simulink model "EM25_Matlab"  (R2024b)
settings: Solver=FixedStepAuto  StartTime=0.0  StopTime=0.5  RelTol=1e-3
libraries: spsRMSLib x10, spsThreePhaseVIMeasurementLib x6, spsGroundLib x6, spsThreePhaseTransformerTwoWindingsLib x5, eePowerMeasurement x5, spsThreePhaseParallelRLCBranchLib x4, spsThreePhaseBreakerLib x4, spsSynchronousMachinepuStandardLib x3, spsThreePhasePISectionLineLib x1, spsThreePhaseSeriesRLCLoadLib x1, sps_lib x1
settings Model: Creator=User  LastModifiedBy=User

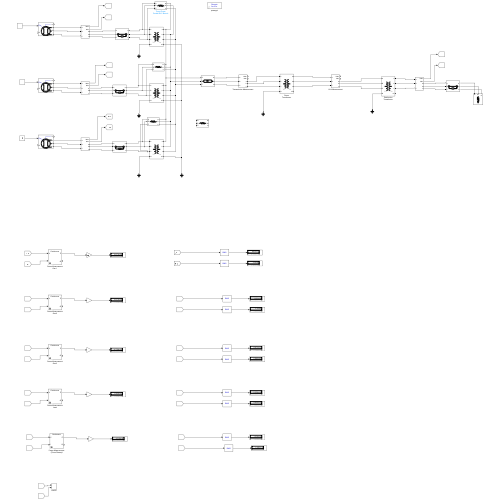
[thumbnail: Simulink's stored preview of the top-level diagram]
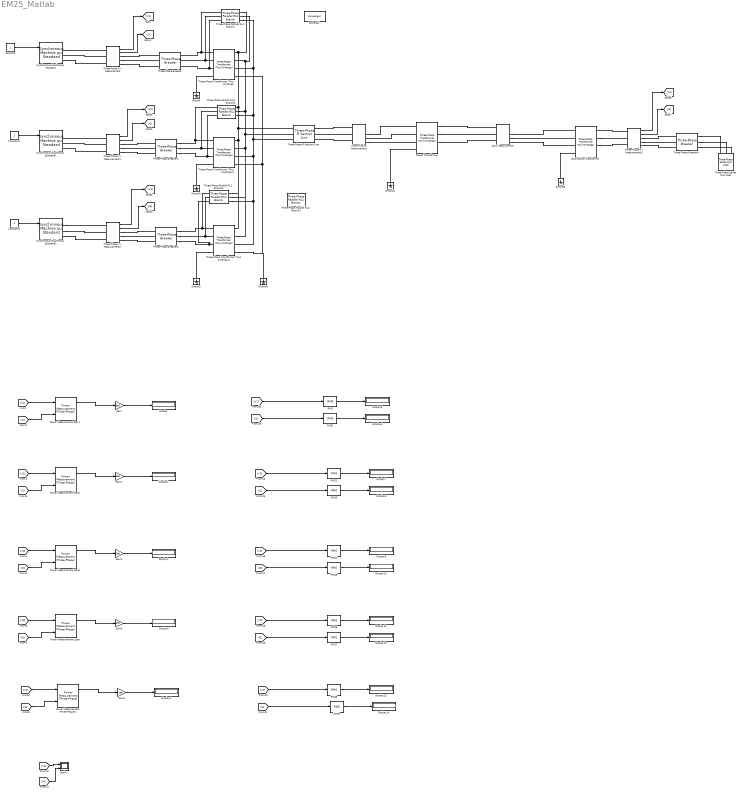
== system EM25_Matlab ==
  11kV Measurement : spsThreePhaseVIMeasurementLib/Three-Phase V-I Measurement  VoltageMeasurement=phase-to-ground  SetLabelV=off  LabelV=Vabc  Vpu=off  VpuLL=off  CurrentMeasurement=yes  SetLabelI=off  LabelI=Iabc  Ipu=off  Pbase=100e6  Vbase=500e3  OutputType=Complex  PhasorSimulation=off  PSBequivalent=0
  Constant : Constant
  Constant1 : Constant
  Constant2 : Constant
  Display{,1..14} (15 alike) : Display
  Distribution Transformer : spsThreePhaseTransformerTwoWindingsLib/Three-Phase Transformer (Two Windings)  Winding1Connection=Yn  Winding2Connection=Yn  CoreType=Three single-phase transformers  SetSaturation=off  Hysteresis=off  DataFile='hysteresis'  SetInitialFlux=off  Measurements=None  UNITS=pu  NominalPower=[ 3e6 , 50 ]  Winding1=[ 11000 , 0.01 , 0.05 ]  Winding2=[ 400 , 0.01 , 0.05 ]  Rm=500  Lm=500  L0=0.5  Saturation=[ 0,0 ; 0.0024,1.2 ; 1.0,1.52 ]  InitialFluxes=[ 0.8 , -0.8 , 0.7 ]  BreakLoop=off  DiscreteSolver=Trapezoidal iterative  DataType=off  TransfoNumber=1
  Gain{,1..4} (5 alike) : Gain  Gain=1e6
  Ground{,1..5} (6 alike) : spsGroundLib/Ground  LConnTagsString=a
  Power Transformer : spsThreePhaseTransformerTwoWindingsLib/Three-Phase Transformer (Two Windings)  Winding1Connection=Yn  Winding2Connection=Yn  CoreType=Three single-phase transformers  SetSaturation=off  Hysteresis=off  DataFile='hysteresis'  SetInitialFlux=off  Measurements=None  UNITS=pu  NominalPower=[ 10e6 , 50 ]  Winding1=[ 132000 , 0.002 , 0.08 ]  Winding2=[ 11000 , 0.002 , 0.08 ]  Rm=500  Lm=500  L0=0.5  Saturation=[ 0,0 ; 0.0024,1.2 ; 1.0,1.52 ]  InitialFluxes=[ 0.8 , -0.8 , 0.7 ]  BreakLoop=off  DiscreteSolver=Trapezoidal iterative  DataType=off  TransfoNumber=1
  Power Measurement (Three-Phase)4 : eePowerMeasurement/Power Measurement (Three-Phase)  LabelModeActiveChoice=Continuous  F=50  K=[0 1 2 3]  Seq=Positive  Ts=0
  Power Measurement Gen 1 : eePowerMeasurement/Power Measurement (Three-Phase)  LabelModeActiveChoice=Continuous  F=50  K=[0 1 2 3]  Seq=Positive  Ts=0
  Power Measurement Gen2 : eePowerMeasurement/Power Measurement (Three-Phase)  LabelModeActiveChoice=Continuous  F=50  K=[0 1 2 3]  Seq=Positive  Ts=0
  Power Measurement Gen3 : eePowerMeasurement/Power Measurement (Three-Phase)  LabelModeActiveChoice=Continuous  F=50  K=[0 1 2 3]  Seq=Positive  Ts=0
  Power Measurement Load : eePowerMeasurement/Power Measurement (Three-Phase)  LabelModeActiveChoice=Continuous  F=50  K=[0 1 2 3]  Seq=Positive  Ts=0
  RMS{,1..9} (10 alike) : spsRMSLib/RMS  TrueRMS=on  Freq=60  RMSInit=120  Ts=0
  Synchronous Machine pu Standard : spsSynchronousMachinepuStandardLib/Synchronous Machine pu Standard  PresetModel=No  MechanicalLoad=Mechanical power Pm  ShowDetailedParameters=on  RotorType=Round  Units=per unit standard parameters  MeasurementBus=off  NominalParameters=[1e6 11000 50]  Reactances1=[ 1.81, 0.3, 0.23, 1.76, 0.65, 0.25, 0.15 ]  Reactances2=[2.24 0.17 0.12 1.02 0.13 0.08]  dAxisTimeConstants=Short-circuit  qAxisTimeConstants=Short-circuit  TimeConstants1="[ 4.4849  0.0681  0.1  ]"  TimeConstants2=[ 8.0, 0.03, 1.0, 0.07 ]  TimeConstants3="[  4.49  0.0681  0.0513  ]"  TimeConstants4=[ 8.0, 0.03, 0.3371, 0.0295 ]  TimeConstants5=[ 1.01, 0.053, 0.1 ]  TimeConstants6=[ 1.3201, 0.023, 1.0, 0.07 ]  TimeConstants7=[0.012 0.003 0.003]  TimeConstants8=[ 1.3201, 0.0231, 0.3371, 0.0295 ]  StatorResistance=0.005  Mechanical=[3 0.01 2]  PolePairs=20  InitialConditions="[ 0  0  0  0  0  0  0  0  1 ]"  SetSaturation=off  Saturation=[0.6404,0.7127,0.8441,0.9214,0.9956,1.082,1.19,1.316,1.457;0.7,0.7698,0.8872,0.9466,0.9969,1.046,1.1,1.151,1.201]  LoadFlowParameters=[1,0,0,0,0]  TsPowergui=0  TsBlock=-1  IterativeModel=Trapezoidal non iterative  IterativeDiscreteModel=Trapezoidal non iterative  BusType=PV  Pref=0  Qref=0  Qmin=-inf  Qmax=inf  PLF=0  QLF=0
  Synchronous Machine pu Standard1 : spsSynchronousMachinepuStandardLib/Synchronous Machine pu Standard  PresetModel=No  MechanicalLoad=Mechanical power Pm  ShowDetailedParameters=on  RotorType=Round  Units=per unit standard parameters  MeasurementBus=off  NominalParameters=[2e6 12000 50]  Reactances1=[ 1.81, 0.3, 0.23, 1.76, 0.65, 0.25, 0.15 ]  Reactances2=[2.24 0.17 0.12 1.02 0.13 0.08]  dAxisTimeConstants=Short-circuit  qAxisTimeConstants=Short-circuit  TimeConstants1="[ 4.4849  0.0681  0.1  ]"  TimeConstants2=[ 8.0, 0.03, 1.0, 0.07 ]  TimeConstants3="[  4.49  0.0681  0.0513  ]"  TimeConstants4=[ 8.0, 0.03, 0.3371, 0.0295 ]  TimeConstants5=[ 1.01, 0.053, 0.1 ]  TimeConstants6=[ 1.3201, 0.023, 1.0, 0.07 ]  TimeConstants7=[0.012 0.003 0.003]  TimeConstants8=[ 1.3201, 0.0231, 0.3371, 0.0295 ]  StatorResistance=0.005  Mechanical=[3 0.01 2]  PolePairs=20  InitialConditions="[ 0  0  0  0  0  0  0  0  1 ]"  SetSaturation=off  Saturation=[0.6404,0.7127,0.8441,0.9214,0.9956,1.082,1.19,1.316,1.457;0.7,0.7698,0.8872,0.9466,0.9969,1.046,1.1,1.151,1.201]  LoadFlowParameters=[1,0,0,0,0]  TsPowergui=0  TsBlock=-1  IterativeModel=Trapezoidal non iterative  IterativeDiscreteModel=Trapezoidal non iterative  BusType=PV  Pref=0  Qref=0  Qmin=-inf  Qmax=inf  PLF=0  QLF=0
  Synchronous Machine pu Standard2 : spsSynchronousMachinepuStandardLib/Synchronous Machine pu Standard  PresetModel=No  MechanicalLoad=Mechanical power Pm  ShowDetailedParameters=on  RotorType=Round  Units=per unit standard parameters  MeasurementBus=off  NominalParameters=[4e6 10000 50]  Reactances1=[ 1.81, 0.3, 0.23, 1.76, 0.65, 0.25, 0.15 ]  Reactances2=[2.24 0.17 0.12 1.02 0.13 0.08]  dAxisTimeConstants=Short-circuit  qAxisTimeConstants=Short-circuit  TimeConstants1="[ 4.4849  0.0681  0.1  ]"  TimeConstants2=[ 8.0, 0.03, 1.0, 0.07 ]  TimeConstants3="[  4.49  0.0681  0.0513  ]"  TimeConstants4=[ 8.0, 0.03, 0.3371, 0.0295 ]  TimeConstants5=[ 1.01, 0.053, 0.1 ]  TimeConstants6=[ 1.3201, 0.023, 1.0, 0.07 ]  TimeConstants7=[0.012 0.003 0.003]  TimeConstants8=[ 1.3201, 0.0231, 0.3371, 0.0295 ]  StatorResistance=0.005  Mechanical=[3 0.01 2]  PolePairs=20  InitialConditions="[ 0  0  0  0  0  0  0  0  1 ]"  SetSaturation=off  Saturation=[0.6404,0.7127,0.8441,0.9214,0.9956,1.082,1.19,1.316,1.457;0.7,0.7698,0.8872,0.9466,0.9969,1.046,1.1,1.151,1.201]  LoadFlowParameters=[1,0,0,0,0]  TsPowergui=0  TsBlock=-1  IterativeModel=Trapezoidal non iterative  IterativeDiscreteModel=Trapezoidal non iterative  BusType=PV  Pref=0  Qref=0  Qmin=-inf  Qmax=inf  PLF=0  QLF=0
  Three-Phase PI Section Line : spsThreePhasePISectionLineLib/Three-Phase PI Section Line  LConnTagsString=a|b|c  RConnTagsString=A|B|C  Length=50  Frequency=50  Resistances=[ 0.05 0.15]  Inductances="[ 1e-3  3e-3]"  Capacitances=[1e-8 5e-9]
  Three-Phase Parallel RLC Branch{,1..3} (4 alike) : spsThreePhaseParallelRLCBranchLib/Three-Phase Parallel RLC Branch  LConnTagsString=A|B|C  RConnTagsString=A|B|C  BranchType=R  Resistance=1E6  Inductance=0  Capacitance=0  Measurements=None
  Three-Phase Series RLC Load : spsThreePhaseSeriesRLCLoadLib/Three-Phase Series RLC Load  LConnTagsString=A|B|C  Configuration=Y (grounded)  NominalVoltage=400  Vabc=[1e3 1e3 1e3]  Vabcp=[1e3 1e3 1e3]  NominalFrequency=50  UnbalancedPower=off  ActivePower=2e6  InductivePower=0  CapacitivePower=0  Pabc=[10e3 9e3 11e3]  QLabc=[100 90 110]  QCabc=[100 90 110]  Pabcp=[10e3 9e3 11e3]  QLabcp=[100 90 110]  QCabcp=[100 90 110]  Measurements=None  LoadType=constant Z
  Three-Phase Transformer (Two Windings) : spsThreePhaseTransformerTwoWindingsLib/Three-Phase Transformer (Two Windings)  Winding1Connection=Yn  Winding2Connection=Yn  CoreType=Three single-phase transformers  SetSaturation=off  Hysteresis=off  DataFile='hysteresis'  SetInitialFlux=off  Measurements=None  UNITS=pu  NominalPower=[ 1e6 , 50 ]  Winding1=[ 11000 , 0.002 , 0.08 ]  Winding2=[ 132000 , 0.002 , 0.08 ]  Rm=500  Lm=500  L0=0.5  Saturation=[ 0,0 ; 0.0024,1.2 ; 1.0,1.52 ]  InitialFluxes=[ 0.8 , -0.8 , 0.7 ]  BreakLoop=off  DiscreteSolver=Trapezoidal iterative  DataType=off  TransfoNumber=1
  Three-Phase Transformer (Two Windings)1 : spsThreePhaseTransformerTwoWindingsLib/Three-Phase Transformer (Two Windings)  Winding1Connection=Yn  Winding2Connection=Yn  CoreType=Three single-phase transformers  SetSaturation=off  Hysteresis=off  DataFile='hysteresis'  SetInitialFlux=off  Measurements=None  UNITS=pu  NominalPower=[ 2e6 , 50 ]  Winding1=[ 12000 , 0.002 , 0.08 ]  Winding2=[ 132000 , 0.002 , 0.08 ]  Rm=500  Lm=500  L0=0.5  Saturation=[ 0,0 ; 0.0024,1.2 ; 1.0,1.52 ]  InitialFluxes=[ 0.8 , -0.8 , 0.7 ]  BreakLoop=off  DiscreteSolver=Trapezoidal iterative  DataType=off  TransfoNumber=1
  Three-Phase Transformer (Two Windings)2 : spsThreePhaseTransformerTwoWindingsLib/Three-Phase Transformer (Two Windings)  Winding1Connection=Yn  Winding2Connection=Yn  CoreType=Three single-phase transformers  SetSaturation=off  Hysteresis=off  DataFile='hysteresis'  SetInitialFlux=off  Measurements=None  UNITS=pu  NominalPower=[ 4e6 , 50 ]  Winding1=[ 10000 , 0.002 , 0.08 ]  Winding2=[ 132000 , 0.002 , 0.08 ]  Rm=500  Lm=500  L0=0.5  Saturation=[ 0,0 ; 0.0024,1.2 ; 1.0,1.52 ]  InitialFluxes=[ 0.8 , -0.8 , 0.7 ]  BreakLoop=off  DiscreteSolver=Trapezoidal iterative  DataType=off  TransfoNumber=1
  Three-Phase V-I Measurement{,1..3} (4 alike) : spsThreePhaseVIMeasurementLib/Three-Phase V-I Measurement  VoltageMeasurement=phase-to-ground  SetLabelV=off  LabelV=Vabc  Vpu=off  VpuLL=off  CurrentMeasurement=yes  SetLabelI=off  LabelI=Iabc  Ipu=off  Pbase=100e6  Vbase=500e3  OutputType=Complex  PhasorSimulation=off  PSBequivalent=0
  Three-Phase Breaker{,1..2,4} (4 alike) : spsThreePhaseBreakerLib/Three-Phase Breaker  InitialState=closed  SwitchA=on  SwitchB=on  SwitchC=on  SwitchTimes="[1/60  5/60]"  External=off  BreakerResistance=0.001  SnubberResistance=1e5  SnubberCapacitance=inf  Measurements=None
  Transmission Measurement : spsThreePhaseVIMeasurementLib/Three-Phase V-I Measurement  VoltageMeasurement=phase-to-ground  SetLabelV=off  LabelV=Vabc  Vpu=off  VpuLL=off  CurrentMeasurement=yes  SetLabelI=off  LabelI=Iabc  Ipu=off  Pbase=100e6  Vbase=500e3  OutputType=Complex  PhasorSimulation=off  PSBequivalent=0
  load VI : Scope  NumInputPorts=2
  powergui : sps_lib/powergui  Priority=1  SimulationMode=Discrete  SampleTime=50e-6  frequency=60  Iterations=50  frequencyindice=50  Pbase=100e6  ErrMax=1e-4  UnitsV=kV  UnitsW=MW  buscounter=0  FunctionMessages=off  echomessages=off  EnableUseOfTLC=off  CurrentSourceSwitches=off  DisableSnubberDevices=off  DisableRonSwitches=off  DisableVfSwitches=off  DisplayEquations=off  AutomaticDiscreteSolvers=off  SolverType=Tustin/Backward Euler (TBE)  Interpol=off  ExternalGateDelay=off  methode=off  Ts=100  x0status=blocks  SPID=on  SwTol=0  HookPort=off  NonlinearTolerance=1e-4  nMaxIteration=100  ContinueOnMaxIteration=off  RestoreLinks=warning  ResistiveCurrentMeasurement=off  Frange=[0:2:500]  Ylog=off  Xlog=on  ShowGrid=off  save=off  variable=ZData  structure=0  ZoomFFT=off  StartTime=0.0  cycles=1  DisplayStyle=1  fundamental=60  FreqAxis=off  MaxFrequency=1000  frequencyindicesteady=1  RmsSteady=1  display=off
  wires:
  Constant/1 -> Synchronous Machine pu Standard/1
  Constant1/1 -> Synchronous Machine pu Standard1/1
  Constant2/1 -> Synchronous Machine pu Standard2/1
  Three-Phase V-I Measurement/1 -> [V1]
  Three-Phase V-I Measurement/2 -> [I1]
  Three-Phase V-I Measurement1/1 -> [V2]
  Three-Phase V-I Measurement1/2 -> [I2]
  Three-Phase V-I Measurement2/1 -> [V3]
  Three-Phase V-I Measurement2/2 -> [I3]
  [V1] -> Power Measurement Gen 1/1
  [I1] -> Power Measurement Gen 1/2
  Power Measurement Gen 1/1 -> Gain/1
  Gain/1 -> Display/1
  [V1] -> Power Measurement Gen2/1
  [I1] -> Power Measurement Gen2/2
  Gain1/1 -> Display1/1
  Power Measurement Gen2/1 -> Gain1/1
  [V2] -> Power Measurement Gen3/1
  [I2] -> Power Measurement Gen3/2
  Gain2/1 -> Display2/1
  Power Measurement Gen3/1 -> Gain2/1
  [V3] -> Power Measurement Load/1
  [I3] -> Power Measurement Load/2
  Gain3/1 -> Display3/1
  Power Measurement Load/1 -> Gain3/1
  [V4] -> Power Measurement (Three-Phase)4/1
  [I4] -> Power Measurement (Three-Phase)4/2
  Gain4/1 -> Display4/1
  Power Measurement (Three-Phase)4/1 -> Gain4/1
  Three-Phase V-I Measurement3/1 -> [V4]
  Three-Phase V-I Measurement3/2 -> [I4]
  [V4] -> load VI/1
  [I4] -> load VI/2
  [V1] -> RMS/1
  RMS/1 -> Display5/1
  [I1] -> RMS1/1
  RMS1/1 -> Display6/1
  [V1] -> RMS2/1
  RMS2/1 -> Display7/1
  [I1] -> RMS3/1
  RMS3/1 -> Display8/1
  [V2] -> RMS4/1
  RMS4/1 -> Display9/1
  [I2] -> RMS5/1
  RMS5/1 -> Display10/1
  [V3] -> RMS6/1
  RMS6/1 -> Display11/1
  [I3] -> RMS7/1
  RMS7/1 -> Display12/1
  RMS8/1 -> Display13/1
  [V4] -> RMS8/1
  [I4] -> RMS9/1
  RMS9/1 -> Display14/1
  connections:
  Three-Phase V-I Measurement/LConn2 -- Synchronous Machine pu Standard/RConn2
  Synchronous Machine pu Standard/RConn3 -- Three-Phase V-I Measurement/LConn3
  Synchronous Machine pu Standard/RConn1 -- Three-Phase V-I Measurement/LConn1
  Three-Phase V-I Measurement/RConn1 -- Three-Phase Breaker/LConn1
  Three-Phase Transformer (Two Windings)/LConn4 -- Ground/LConn1
  Three-Phase V-I Measurement1/LConn1 -- Synchronous Machine pu Standard1/RConn1
  Three-Phase V-I Measurement1/LConn2 -- Synchronous Machine pu Standard1/RConn2
  Three-Phase V-I Measurement1/LConn3 -- Synchronous Machine pu Standard1/RConn3
  Synchronous Machine pu Standard2/RConn1 -- Three-Phase V-I Measurement2/LConn1
  Synchronous Machine pu Standard2/RConn2 -- Three-Phase V-I Measurement2/LConn2
  Synchronous Machine pu Standard2/RConn3 -- Three-Phase V-I Measurement2/LConn3
  Three-Phase V-I Measurement1/RConn1 -- Three-Phase Breaker1/LConn1
  Three-Phase V-I Measurement1/RConn2 -- Three-Phase Breaker1/LConn2
  Three-Phase V-I Measurement1/RConn3 -- Three-Phase Breaker1/LConn3
  Three-Phase V-I Measurement2/RConn1 -- Three-Phase Breaker2/LConn1
  Three-Phase V-I Measurement2/RConn2 -- Three-Phase Breaker2/LConn2
  Three-Phase V-I Measurement2/RConn3 -- Three-Phase Breaker2/LConn3
  Three-Phase Transformer (Two Windings)1/LConn4 -- Ground1/LConn1
  Three-Phase Transformer (Two Windings)2/LConn4 -- Ground2/LConn1
  Three-Phase Transformer (Two Windings)/RConn1 -- Three-Phase Parallel RLC Branch/RConn1 -- Three-Phase Parallel RLC Branch2/RConn1 -- Three-Phase PI Section Line/LConn1 -- Three-Phase Parallel RLC Branch3/RConn1 -- Three-Phase Transformer (Two Windings)2/RConn1 -- Three-Phase Transformer (Two Windings)1/RConn1
  Three-Phase Transformer (Two Windings)/RConn2 -- Three-Phase Parallel RLC Branch/RConn2 -- Three-Phase Parallel RLC Branch2/RConn2 -- Three-Phase PI Section Line/LConn2 -- Three-Phase Parallel RLC Branch3/RConn2 -- Three-Phase Transformer (Two Windings)2/RConn2 -- Three-Phase Transformer (Two Windings)1/RConn2
  Three-Phase Transformer (Two Windings)/RConn3 -- Three-Phase Parallel RLC Branch/RConn3 -- Three-Phase Parallel RLC Branch2/RConn3 -- Three-Phase PI Section Line/LConn3 -- Three-Phase Transformer (Two Windings)1/RConn3 -- Three-Phase Transformer (Two Windings)2/RConn3 -- Three-Phase Parallel RLC Branch3/RConn3
  Three-Phase Transformer (Two Windings)/RConn4 -- Ground3/LConn1 -- Three-Phase Transformer (Two Windings)2/RConn4 -- Three-Phase Transformer (Two Windings)1/RConn4
  Three-Phase PI Section Line/RConn1 -- Transmission Measurement/LConn1
  Transmission Measurement/LConn2 -- Three-Phase PI Section Line/RConn2
  Transmission Measurement/LConn3 -- Three-Phase PI Section Line/RConn3
  Power Transformer/LConn2 -- Transmission Measurement/RConn2
  Transmission Measurement/RConn1 -- Power Transformer/LConn1
  Transmission Measurement/RConn3 -- Power Transformer/LConn3
  Power Transformer/RConn1 -- 11kV Measurement/LConn1
  Power Transformer/RConn2 -- 11kV Measurement/LConn2
  Power Transformer/RConn3 -- 11kV Measurement/LConn3
  Ground4/LConn1 -- Power Transformer/LConn4
  11kV Measurement/RConn1 -- Distribution Transformer/LConn1
  11kV Measurement/RConn2 -- Distribution Transformer/LConn2
  11kV Measurement/RConn3 -- Distribution Transformer/LConn3
  Three-Phase V-I Measurement3/LConn1 -- Distribution Transformer/RConn1
  Distribution Transformer/RConn2 -- Three-Phase V-I Measurement3/LConn2
  Distribution Transformer/RConn3 -- Three-Phase V-I Measurement3/LConn3
  Ground5/LConn1 -- Distribution Transformer/LConn4
  Three-Phase V-I Measurement3/RConn1 -- Three-Phase Breaker4/LConn1
  Three-Phase V-I Measurement3/RConn2 -- Three-Phase Breaker4/LConn2
  Three-Phase V-I Measurement3/RConn3 -- Three-Phase Breaker4/LConn3
  Three-Phase V-I Measurement/RConn2 -- Three-Phase Breaker/LConn2
  Three-Phase V-I Measurement/RConn3 -- Three-Phase Breaker/LConn3
  Three-Phase Transformer (Two Windings)/LConn1 -- Three-Phase Parallel RLC Branch/LConn1 -- Three-Phase Breaker/RConn1
  Three-Phase Transformer (Two Windings)/LConn2 -- Three-Phase Parallel RLC Branch/LConn2 -- Three-Phase Breaker/RConn2
  Three-Phase Transformer (Two Windings)/LConn3 -- Three-Phase Parallel RLC Branch/LConn3 -- Three-Phase Breaker/RConn3
  Three-Phase Breaker1/RConn1 -- Three-Phase Parallel RLC Branch2/LConn1 -- Three-Phase Transformer (Two Windings)1/LConn1
  Three-Phase Breaker1/RConn2 -- Three-Phase Parallel RLC Branch2/LConn2 -- Three-Phase Transformer (Two Windings)1/LConn2
  Three-Phase Breaker1/RConn3 -- Three-Phase Parallel RLC Branch2/LConn3 -- Three-Phase Transformer (Two Windings)1/LConn3
  Three-Phase Breaker2/RConn1 -- Three-Phase Parallel RLC Branch3/LConn1 -- Three-Phase Transformer (Two Windings)2/LConn1
  Three-Phase Breaker2/RConn2 -- Three-Phase Parallel RLC Branch3/LConn2 -- Three-Phase Transformer (Two Windings)2/LConn2
  Three-Phase Breaker2/RConn3 -- Three-Phase Parallel RLC Branch3/LConn3 -- Three-Phase Transformer (Two Windings)2/LConn3
  Three-Phase Breaker4/RConn1 -- Three-Phase Series RLC Load/LConn1
  Three-Phase Breaker4/RConn2 -- Three-Phase Series RLC Load/LConn2
  Three-Phase Breaker4/RConn3 -- Three-Phase Series RLC Load/LConn3
